simulink model "mchp_acim_dsPIC33A"  (R2025b)
settings: Solver=FixedStepDiscrete  StartTime=0.0  StopTime=25  FixedStep=Ts  RelTol=1e-3  EnableMultiTasking=on
values from neighbouring files (symbols this model uses):
  dataType = 'single'    [mchp_acim_foc_dsPIC33A_data.m]
  PWM_frequency = 20e3    (= 20000)    [mchp_acim_foc_dsPIC33A_data.m]
  PWM_frequency_mc = PWM_frequency    (= 20000)    [mchp_acim_foc_dsPIC33A_data.m]
  SpeedFilterCutoff = 40    [mchp_acim_foc_dsPIC33A_data.m]
  Ts = T_pwm    (= 5e-05)    [mchp_acim_foc_dsPIC33A_data.m]
  Ts_mc = T_pwm_mc    (= 5e-05)    [mchp_acim_foc_dsPIC33A_data.m]
  Ts_motor = T_pwm_mc    (= 5e-05)    [mchp_acim_foc_dsPIC33A_data.m]
  Ts_serialIn = 100e-3    (= 0.1)    [mchp_acim_foc_dsPIC33A_data.m]
undefined symbols (not defined in the file or in its folder): A0, A4, acim, ADC, appState, B0, C10, C11, C6, C7, C8, CS_param, D11, D12, DiscIntNeverNeededParam, estim_pll, estim_qei, inverter, Max, MaxPer, ms, NumBits1, NumBits2, P1, P17, P20, P39, P40, P41, P43, P44, P60, P61, PI_params_SI, Pin, PWM4_Trg1, Resol, s, target, us, VmaxPhase
libraries: simulink x47, MCHP_Blockset x24, mcbcontrolslib x5, mcbeeMathTransformLib x4, slpidlib x4, svdutilitieslib x1, autolibim x1, mcbplantlib x1
(part 4 of 6)

== system mchp_acim_dsPIC33A/MCHV-230VAC-1.5kW Development Board dsPIC33AK128MC106 MC DIM/ADC ==
  ADC HS 12b dsPICA : MCHP_Blockset/Analog IO/ADC HS 12b dsPICA  ADCREF=ADC 1 and ADC 2  ADC1_refChannel=0 (highest priority)  ADC2_refChannel=0 (highest priority)  ADC3_refChannel=Not used  ADC4_refChannel=Not used  ADC5_refChannel=Not used  CALRATE=once at startup  VREF_RNG=3.0V to 3.6V  BUFEN=off  info=0  SampleTime=1/Switching_Frequency  MCHP_PORT={ADC1_seq0.0}{ADC1A7}15:2:A7;{ADC2_seq0.0}{ADC2B7}15:2:B7;{ADC1_seq0.1}{ADC1B6}15:2:B6;{ADC1_seq0.0}{ADC1A7}15:2:A7;{ADC2_seq0.0}{ADC2B7}15:2:B7;{ADC1_seq0.1}{ADC1B6}15:2:B6;  MCHP_MASTERLINK=mchp_acim_dsPIC33A/MCHV-230VAC-1.5kW Development Board dsPIC33AK128MC106 MC DIM/Microchip Master  MCHP_CRC=33524962  ADC_Synchronisation=Triggered by custom source  ADC_Trig_TXT=PWM4_Trg1  ADC_TrigTimeStep=on  TrigSource_seq0_TXT=PWM4 adc trig 1  SampleTime_seq0_Tad_TXT="8.5 Tad  = 106ns  -  Rin < 11 kOhm"  ADC1_seq0_TXT=AD1 AN6 / A7 / Pin[2]  ADC1_seq0_align=Left aligned  ADC1_seq0_overSampling=x1 (12 bits)  ADC2_seq0_TXT=AD2 AN8 / B7 / Pin[30]  ADC2_seq0_align=Right aligned  ADC2_seq0_overSampling=x1 (12 bits)  ADC3_seq0_TXT="AD2 AN1 / B0 / Pin[20]  (L)"  ADC3_seq0_align=Right aligned  ADC3_seq0_overSampling=x1 (12 bits)  ADC4_seq0_TXT="AD2 AN1 / B0 / Pin[20]  (L)"  ADC4_seq0_align=Right aligned  ADC4_seq0_overSampling=x1 (12 bits)  ADC5_seq0_TXT="AD2 AN1 / B0 / Pin[20]  (L)"  ADC5_seq0_align=Right aligned  ADC5_seq0_overSampling=x1 (12 bits)  ADC1_seq0_1_TXT=AD1 AN8 / B6 / Pin[29]  ADC1_seq0_1_align=Left aligned  ADC1_seq0_1_overSampling=x1 (12 bits)  ADC2_seq0_1_TXT=Not Used  ADC2_seq0_1_align=Right aligned  ADC2_seq0_1_overSampling=x1 (12 bits)  ADC3_seq0_1_TXT=Not Used  ADC3_seq0_1_align=Right aligned  ADC3_seq0_1_overSampling=x1 (12 bits)  ADC4_seq0_1_TXT=Not Used  ADC4_seq0_1_align=Right aligned  ADC4_seq0_1_overSampling=x1 (12 bits)  ADC5_seq0_1_TXT=Not Used  ADC5_seq0_1_align=Right aligned  ADC5_seq0_1_overSampling=x1 (12 bits)  ADC1_seq0_2_TXT=Not Used  ADC1_seq0_2_align=Right aligned  ADC1_seq0_2_overSampling=x1 (12 bits)  ADC2_seq0_2_TXT=Not Used  ADC2_seq0_2_align=Right aligned  ADC2_seq0_2_overSampling=x1 (12 bits)  ADC3_seq0_2_TXT=Not Used  ADC3_seq0_2_align=Right aligned  ADC3_seq0_2_overSampling=x1 (12 bits)  ADC4_seq0_2_TXT=Not Used  ADC4_seq0_2_align=Right aligned  ADC4_seq0_2_overSampling=x1 (12 bits)  ADC5_seq0_2_TXT=Not Used  ADC5_seq0_2_align=Right aligned  ADC5_seq0_2_overSampling=x1 (12 bits)  ADC1_seq0_3_TXT=Not Used  ADC1_seq0_3_align=Right aligned  ADC1_seq0_3_overSampling=x1 (12 bits)  ADC2_seq0_3_TXT=Not Used  ADC2_seq0_3_align=Right aligned  ADC2_seq0_3_overSampling=x1 (12 bits)  ADC3_seq0_3_TXT=Not Used  ADC3_seq0_3_align=Right aligned  ADC3_seq0_3_overSampling=x1 (12 bits)  ADC4_seq0_3_TXT=Not Used  ADC4_seq0_3_align=Right aligned  ADC4_seq0_3_overSampling=x1 (12 bits)  ADC5_seq0_3_TXT=Not Used  ADC5_seq0_3_align=Right aligned  ADC5_seq0_3_overSampling=x1 (12 bits)  ADC1_seq0_4_TXT=Not Used  ADC1_seq0_4_align=Right aligned  ADC1_seq0_4_overSampling=x1 (12 bits)  ADC2_seq0_4_TXT=Not Used  ADC2_seq0_4_align=Right aligned  ADC2_seq0_4_overSampling=x1 (12 bits)  ADC3_seq0_4_TXT=Not Used  ADC3_seq0_4_align=Right aligned  ADC3_seq0_4_overSampling=x1 (12 bits)  ADC4_seq0_4_TXT=Not Used  ADC4_seq0_4_align=Right aligned  ADC4_seq0_4_overSampling=x1 (12 bits)  ADC5_seq0_4_TXT=Not Used  ADC5_seq0_4_align=Right aligned  ADC5_seq0_4_overSampling=x1 (12 bits)  ADC1_seq0_5_TXT=Not Used  ADC1_seq0_5_align=Right aligned  ADC1_seq0_5_overSampling=x1 (12 bits)  ADC2_seq0_5_TXT=Not Used  ADC2_seq0_5_align=Right aligned  ADC2_seq0_5_overSampling=x1 (12 bits)  ADC3_seq0_5_TXT=Not Used  ADC3_seq0_5_align=Right aligned  ADC3_seq0_5_overSampling=x1 (12 bits)  ADC4_seq0_5_TXT=Not Used  ADC4_seq0_5_align=Right aligned  ADC4_seq0_5_overSampling=x1 (12 bits)  ADC5_seq0_5_TXT=Not Used  ADC5_seq0_5_align=Right aligned  ADC5_seq0_5_overSampling=x1 (12 bits)  ADC_TRG2_ACCBRST_seq0=Burst - not interruptible  ADC1_NINSEL_seq0_TXT=Vss - single ended (unsigned)  ADC2_NINSEL_seq0_TXT=Vss - single ended (unsigned)  ADC3_NINSEL_seq0_TXT=Vss - single ended (unsigned)  ADC4_NINSEL_seq0_TXT=Vss - single ended (unsigned)  ADC5_NINSEL_seq0_TXT=Vss - single ended (unsigned)  TrigTimeStep_seq0=on  info_seq0=0  TrigSource_seq1_TXT=after previous sequence  SampleTime_seq1_Tad_TXT="4.5 Tad  = 56.2ns  -  Rin < 5.2 kOhm"  ADC1_seq1_TXT=Not Used  ADC1_seq1_align=Left aligned  ADC1_seq1_overSampling=x1 (12 bits)  ADC2_seq1_TXT=Not Used  ADC2_seq1_align=Right aligned  ADC2_seq1_overSampling=x1 (12 bits)  ADC3_seq1_TXT="AD2 AN1 / B0 / Pin[20]  (L)"  ADC3_seq1_align=Right aligned  ADC3_seq1_overSampling=x1 (12 bits)  ADC4_seq1_TXT="AD2 AN1 / B0 / Pin[20]  (L)"  ADC4_seq1_align=Right aligned  ADC4_seq1_overSampling=x1 (12 bits)  ADC5_seq1_TXT="AD2 AN1 / B0 / Pin[20]  (L)"  ADC5_seq1_align=Right aligned  ADC5_seq1_overSampling=x1 (12 bits)  ADC1_seq1_1_TXT=Not Used  ADC1_seq1_1_align=Right aligned  ADC1_seq1_1_overSampling=x1 (12 bits)  ADC2_seq1_1_TXT=Not Used  ADC2_seq1_1_align=Right aligned  ADC2_seq1_1_overSampling=x1 (12 bits)  ADC3_seq1_1_TXT=Not Used  ADC3_seq1_1_align=Right aligned  ADC3_seq1_1_overSampling=x1 (12 bits)  ADC4_seq1_1_TXT=Not Used  ADC4_seq1_1_align=Right aligned  ADC4_seq1_1_overSampling=x1 (12 bits)  ADC5_seq1_1_TXT=Not Used  ADC5_seq1_1_align=Right aligned  ADC5_seq1_1_overSampling=x1 (12 bits)  ADC1_seq1_2_TXT=Not Used  ADC1_seq1_2_align=Right aligned  ADC1_seq1_2_overSampling=x1 (12 bits)  ADC2_seq1_2_TXT=Not Used  ADC2_seq1_2_align=Right aligned  ADC2_seq1_2_overSampling=x1 (12 bits)  ADC3_seq1_2_TXT=Not Used  ADC3_seq1_2_align=Right aligned  ADC3_seq1_2_overSampling=x1 (12 bits)  ADC4_seq1_2_TXT=Not Used  ADC4_seq1_2_align=Right aligned  ADC4_seq1_2_overSampling=x1 (12 bits)  ADC5_seq1_2_TXT=Not Used  ADC5_seq1_2_align=Right aligned  ADC5_seq1_2_overSampling=x1 (12 bits)  ADC1_seq1_3_TXT=Not Used  ADC1_seq1_3_align=Right aligned  ADC1_seq1_3_overSampling=x1 (12 bits)  ADC2_seq1_3_TXT=Not Used  ADC2_seq1_3_align=Right aligned  ADC2_seq1_3_overSampling=x1 (12 bits)  ADC3_seq1_3_TXT=Not Used  ADC3_seq1_3_align=Right aligned  ADC3_seq1_3_overSampling=x1 (12 bits)  ADC4_seq1_3_TXT=Not Used  ADC4_seq1_3_align=Right aligned  ADC4_seq1_3_overSampling=x1 (12 bits)  ADC5_seq1_3_TXT=Not Used  ADC5_seq1_3_align=Right aligned  ADC5_seq1_3_overSampling=x1 (12 bits)  ADC1_seq1_4_TXT=Not Used  ADC1_seq1_4_align=Right aligned  ADC1_seq1_4_overSampling=x1 (12 bits)  ADC2_seq1_4_TXT=Not Used  ADC2_seq1_4_align=Right aligned  ADC2_seq1_4_overSampling=x1 (12 bits)  ADC3_seq1_4_TXT=Not Used  ADC3_seq1_4_align=Right aligned  ADC3_seq1_4_overSampling=x1 (12 bits)  ADC4_seq1_4_TXT=Not Used  ADC4_seq1_4_align=Right aligned  ADC4_seq1_4_overSampling=x1 (12 bits)  ADC5_seq1_4_TXT=Not Used  ADC5_seq1_4_align=Right aligned  ADC5_seq1_4_overSampling=x1 (12 bits)  ADC1_seq1_5_TXT=Not Used  ADC1_seq1_5_align=Right aligned  ADC1_seq1_5_overSampling=x1 (12 bits)  ADC2_seq1_5_TXT=Not Used  ADC2_seq1_5_align=Right aligned  ADC2_seq1_5_overSampling=x1 (12 bits)  ADC3_seq1_5_TXT=Not Used  ADC3_seq1_5_align=Right aligned  ADC3_seq1_5_overSampling=x1 (12 bits)  ADC4_seq1_5_TXT=Not Used  ADC4_seq1_5_align=Right aligned  ADC4_seq1_5_overSampling=x1 (12 bits)  ADC5_seq1_5_TXT=Not Used  ADC5_seq1_5_align=Right aligned  ADC5_seq1_5_overSampling=x1 (12 bits)  ADC_TRG2_ACCBRST_seq1=Burst - not interruptible  ADC1_NINSEL_seq1_TXT=Vss - single ended (unsigned)  ADC2_NINSEL_seq1_TXT=Vss - single ended (unsigned)  ADC3_NINSEL_seq1_TXT=Vss - single ended (unsigned)  ADC4_NINSEL_seq1_TXT=Vss - single ended (unsigned)  ADC5_NINSEL_seq1_TXT=Vss - single ended (unsigned)  TrigTimeStep_seq1=on  info_seq1=0  TrigSource_seq2_TXT=after previous sequence  SampleTime_seq2_Tad_TXT="4.5 Tad  = 56.2ns  -  Rin < 5.2 kOhm"  ADC1_seq2_TXT=Not Used  ADC1_seq2_align=Left aligned  ADC1_seq2_overSampling=x1 (12 bits)  ADC2_seq2_TXT=Not Used  ADC2_seq2_align=Right aligned  ADC2_seq2_overSampling=x1 (12 bits)  ADC3_seq2_TXT="AD2 AN1 / B0 / Pin[20]  (L)"  ADC3_seq2_align=Right aligned  ADC3_seq2_overSampling=x1 (12 bits)  ADC4_seq2_TXT="AD2 AN1 / B0 / Pin[20]  (L)"  ADC4_seq2_align=Right aligned  ADC4_seq2_overSampling=x1 (12 bits)  ADC5_seq2_TXT="AD2 AN1 / B0 / Pin[20]  (L)"  ADC5_seq2_align=Right aligned  ADC5_seq2_overSampling=x1 (12 bits)  ADC1_seq2_1_TXT=Not Used  ADC1_seq2_1_align=Right aligned  ADC1_seq2_1_overSampling=x1 (12 bits)  ADC2_seq2_1_TXT=Not Used  ADC2_seq2_1_align=Right aligned  ADC2_seq2_1_overSampling=x1 (12 bits)  ADC3_seq2_1_TXT=Not Used  ADC3_seq2_1_align=Right aligned  ADC3_seq2_1_overSampling=x1 (12 bits)  ADC4_seq2_1_TXT=Not Used  ADC4_seq2_1_align=Right aligned  ADC4_seq2_1_overSampling=x1 (12 bits)  ADC5_seq2_1_TXT=Not Used  ADC5_seq2_1_align=Right aligned  ADC5_seq2_1_overSampling=x1 (12 bits)  ADC1_seq2_2_TXT=Not Used  ADC1_seq2_2_align=Right aligned  ADC1_seq2_2_overSampling=x1 (12 bits)  ADC2_seq2_2_TXT=Not Used  ADC2_seq2_2_align=Right aligned  ADC2_seq2_2_overSampling=x1 (12 bits)  ADC3_seq2_2_TXT=Not Used  ADC3_seq2_2_align=Right aligned  ADC3_seq2_2_overSampling=x1 (12 bits)  ADC4_seq2_2_TXT=Not Used  ADC4_seq2_2_align=Right aligned  ADC4_seq2_2_overSampling=x1 (12 bits)  ADC5_seq2_2_TXT=Not Used  ADC5_seq2_2_align=Right aligned  ADC5_seq2_2_overSampling=x1 (12 bits)  ADC1_seq2_3_TXT=Not Used  ADC1_seq2_3_align=Right aligned  ADC1_seq2_3_overSampling=x1 (12 bits)  ADC2_seq2_3_TXT=Not Used  ADC2_seq2_3_align=Right aligned  ADC2_seq2_3_overSampling=x1 (12 bits)  ADC3_seq2_3_TXT=Not Used  ADC3_seq2_3_align=Right aligned  ADC3_seq2_3_overSampling=x1 (12 bits)  ADC4_seq2_3_TXT=Not Used  ADC4_seq2_3_align=Right aligned  ADC4_seq2_3_overSampling=x1 (12 bits)  ADC5_seq2_3_TXT=Not Used  ADC5_seq2_3_align=Right aligned  ADC5_seq2_3_overSampling=x1 (12 bits)  ADC1_seq2_4_TXT=Not Used  ADC1_seq2_4_align=Right aligned  ADC1_seq2_4_overSampling=x1 (12 bits)  ADC2_seq2_4_TXT=Not Used  ADC2_seq2_4_align=Right aligned  ADC2_seq2_4_overSampling=x1 (12 bits)  ADC3_seq2_4_TXT=Not Used  ADC3_seq2_4_align=Right aligned  ADC3_seq2_4_overSampling=x1 (12 bits)  ADC4_seq2_4_TXT=Not Used  ADC4_seq2_4_align=Right aligned  ADC4_seq2_4_overSampling=x1 (12 bits)  ADC5_seq2_4_TXT=Not Used  ADC5_seq2_4_align=Right aligned  ADC5_seq2_4_overSampling=x1 (12 bits)  ADC1_seq2_5_TXT=Not Used  ADC1_seq2_5_align=Right aligned  ADC1_seq2_5_overSampling=x1 (12 bits)  ADC2_seq2_5_TXT=Not Used  ADC2_seq2_5_align=Right aligned  ADC2_seq2_5_overSampling=x1 (12 bits)  ADC3_seq2_5_TXT=Not Used  ADC3_seq2_5_align=Right aligned  ADC3_seq2_5_overSampling=x1 (12 bits)  ADC4_seq2_5_TXT=Not Used  ADC4_seq2_5_align=Right aligned  ADC4_seq2_5_overSampling=x1 (12 bits)  ADC5_seq2_5_TXT=Not Used  ADC5_seq2_5_align=Right aligned  ADC5_seq2_5_overSampling=x1 (12 bits)  ADC_TRG2_ACCBRST_seq2=Burst - not interruptible  ADC1_NINSEL_seq2_TXT=Vss - single ended (unsigned)  ADC2_NINSEL_seq2_TXT=Vss - single ended (unsigned)  ADC3_NINSEL_seq2_TXT=Vss - single ended (unsigned)  ADC4_NINSEL_seq2_TXT=Vss - single ended (unsigned)  ADC5_NINSEL_seq2_TXT=Vss - single ended (unsigned)  TrigTimeStep_seq2=on  info_seq2=0  TrigSource_seq3_TXT=after previous sequence  SampleTime_seq3_Tad_TXT="4.5 Tad  = 56.2ns  -  Rin < 5.2 kOhm"  ADC1_seq3_TXT=Not Used  ADC1_seq3_align=Left aligned  ADC1_seq3_overSampling=x1 (12 bits)  ADC2_seq3_TXT=Not Used  ADC2_seq3_align=Right aligned  ADC2_seq3_overSampling=x1 (12 bits)  ADC3_seq3_TXT="AD2 AN1 / B0 / Pin[20]  (L)"  ADC3_seq3_align=Right aligned  ADC3_seq3_overSampling=x1 (12 bits)  ADC4_seq3_TXT="AD2 AN1 / B0 / Pin[20]  (L)"  ADC4_seq3_align=Right aligned  ADC4_seq3_overSampling=x1 (12 bits)  ADC5_seq3_TXT="AD2 AN1 / B0 / Pin[20]  (L)"  ADC5_seq3_align=Right aligned  ADC5_seq3_overSampling=x1 (12 bits)  ADC1_seq3_1_TXT=Not Used  ADC1_seq3_1_align=Right aligned  ADC1_seq3_1_overSampling=x1 (12 bits)  ADC2_seq3_1_TXT=Not Used  ADC2_seq3_1_align=Right aligned  ADC2_seq3_1_overSampling=x1 (12 bits)  ADC3_seq3_1_TXT=Not Used  ADC3_seq3_1_align=Right aligned  ADC3_seq3_1_overSampling=x1 (12 bits)  ADC4_seq3_1_TXT=Not Used  ADC4_seq3_1_align=Right aligned  ADC4_seq3_1_overSampling=x1 (12 bits)  ADC5_seq3_1_TXT=Not Used  ADC5_seq3_1_align=Right aligned  ADC5_seq3_1_overSampling=x1 (12 bits)  ADC1_seq3_2_TXT=Not Used  ADC1_seq3_2_align=Right aligned  ADC1_seq3_2_overSampling=x1 (12 bits)  ADC2_seq3_2_TXT=Not Used  ADC2_seq3_2_align=Right aligned  ADC2_seq3_2_overSampling=x1 (12 bits)  ADC3_seq3_2_TXT=Not Used  ADC3_seq3_2_align=Right aligned  ADC3_seq3_2_overSampling=x1 (12 bits)  ADC4_seq3_2_TXT=Not Used  ADC4_seq3_2_align=Right aligned  ADC4_seq3_2_overSampling=x1 (12 bits)  ADC5_seq3_2_TXT=Not Used  ADC5_seq3_2_align=Right aligned  ADC5_seq3_2_overSampling=x1 (12 bits)  ADC1_seq3_3_TXT=Not Used  ADC1_seq3_3_align=Right aligned  ADC1_seq3_3_overSampling=x1 (12 bits)  ADC2_seq3_3_TXT=Not Used  ADC2_seq3_3_align=Right aligned  ADC2_seq3_3_overSampling=x1 (12 bits)  ADC3_seq3_3_TXT=Not Used  ADC3_seq3_3_align=Right aligned  ADC3_seq3_3_overSampling=x1 (12 bits)  ADC4_seq3_3_TXT=Not Used  ADC4_seq3_3_align=Right aligned  ADC4_seq3_3_overSampling=x1 (12 bits)  ADC5_seq3_3_TXT=Not Used  ADC5_seq3_3_align=Right aligned  ADC5_seq3_3_overSampling=x1 (12 bits)  ADC1_seq3_4_TXT=Not Used  ADC1_seq3_4_align=Right aligned  ADC1_seq3_4_overSampling=x1 (12 bits)  ADC2_seq3_4_TXT=Not Used  ADC2_seq3_4_align=Right aligned  ADC2_seq3_4_overSampling=x1 (12 bits)  ADC3_seq3_4_TXT=Not Used  ADC3_seq3_4_align=Right aligned  ADC3_seq3_4_overSampling=x1 (12 bits)  ADC4_seq3_4_TXT=Not Used  ADC4_seq3_4_align=Right aligned  ADC4_seq3_4_overSampling=x1 (12 bits)  ADC5_seq3_4_TXT=Not Used  ADC5_seq3_4_align=Right aligned  ADC5_seq3_4_overSampling=x1 (12 bits)  ADC1_seq3_5_TXT=Not Used  ADC1_seq3_5_align=Right aligned  ADC1_seq3_5_overSampling=x1 (12 bits)  ADC2_seq3_5_TXT=Not Used  ADC2_seq3_5_align=Right aligned  ADC2_seq3_5_overSampling=x1 (12 bits)  ADC3_seq3_5_TXT=Not Used  ADC3_seq3_5_align=Right aligned  ADC3_seq3_5_overSampling=x1 (12 bits)  ADC4_seq3_5_TXT=Not Used  ADC4_seq3_5_align=Right aligned  ADC4_seq3_5_overSampling=x1 (12 bits)  ADC5_seq3_5_TXT=Not Used  ADC5_seq3_5_align=Right aligned  ADC5_seq3_5_overSampling=x1 (12 bits)  ADC_TRG2_ACCBRST_seq3=Burst - not interruptible  ADC1_NINSEL_seq3_TXT=Vss - single ended (unsigned)  ADC2_NINSEL_seq3_TXT=Vss - single ended (unsigned)  ADC3_NINSEL_seq3_TXT=Vss - single ended (unsigned)  ADC4_NINSEL_seq3_TXT=Vss - single ended (unsigned)  ADC5_NINSEL_seq3_TXT=Vss - single ended (unsigned)  TrigTimeStep_seq3=on  info_seq3=0  TrigSource_seq4_TXT=after previous sequence  SampleTime_seq4_Tad_TXT="4.5 Tad  = 56.2ns  -  Rin < 5.2 kOhm"  ADC1_seq4_TXT=Not Used  ADC1_seq4_align=Left aligned  ADC1_seq4_overSampling=x1 (12 bits)  ADC2_seq4_TXT=Not Used  ADC2_seq4_align=Right aligned  ADC2_seq4_overSampling=x1 (12 bits)  ADC3_seq4_TXT="AD2 AN1 / B0 / Pin[20]  (L)"  ADC3_seq4_align=Right aligned  ADC3_seq4_overSampling=x1 (12 bits)  ADC4_seq4_TXT="AD2 AN1 / B0 / Pin[20]  (L)"  ADC4_seq4_align=Right aligned  ADC4_seq4_overSampling=x1 (12 bits)  ADC5_seq4_TXT="AD2 AN1 / B0 / Pin[20]  (L)"  ADC5_seq4_align=Right aligned  ADC5_seq4_overSampling=x1 (12 bits)  ADC1_seq4_1_TXT=Not Used  ADC1_seq4_1_align=Right aligned  ADC1_seq4_1_overSampling=x1 (12 bits)  ADC2_seq4_1_TXT=Not Used  ADC2_seq4_1_align=Right aligned  ADC2_seq4_1_overSampling=x1 (12 bits)  ADC3_seq4_1_TXT=Not Used  ADC3_seq4_1_align=Right aligned  ADC3_seq4_1_overSampling=x1 (12 bits)  ADC4_seq4_1_TXT=Not Used  ADC4_seq4_1_align=Right aligned  ADC4_seq4_1_overSampling=x1 (12 bits)  ADC5_seq4_1_TXT=Not Used  ADC5_seq4_1_align=Right aligned  ADC5_seq4_1_overSampling=x1 (12 bits)  ADC1_seq4_2_TXT=Not Used  ADC1_seq4_2_align=Right aligned  ADC1_seq4_2_overSampling=x1 (12 bits)  ADC2_seq4_2_TXT=Not Used  ADC2_seq4_2_align=Right aligned  ADC2_seq4_2_overSampling=x1 (12 bits)  ADC3_seq4_2_TXT=Not Used  ADC3_seq4_2_align=Right aligned  ADC3_seq4_2_overSampling=x1 (12 bits)  ADC4_seq4_2_TXT=Not Used  ADC4_seq4_2_align=Right aligned  ADC4_seq4_2_overSampling=x1 (12 bits)  ADC5_seq4_2_TXT=Not Used  ADC5_seq4_2_align=Right aligned  ADC5_seq4_2_overSampling=x1 (12 bits)  ADC1_seq4_3_TXT=Not Used  ADC1_seq4_3_align=Right aligned  ADC1_seq4_3_overSampling=x1 (12 bits)  ADC2_seq4_3_TXT=Not Used  ADC2_seq4_3_align=Right aligned  ADC2_seq4_3_overSampling=x1 (12 bits)  ADC3_seq4_3_TXT=Not Used  ADC3_seq4_3_align=Right aligned  ADC3_seq4_3_overSampling=x1 (12 bits)  ADC4_seq4_3_TXT=Not Used  ADC4_seq4_3_align=Right aligned  ADC4_seq4_3_overSampling=x1 (12 bits)  ADC5_seq4_3_TXT=Not Used  ADC5_seq4_3_align=Right aligned  ADC5_seq4_3_overSampling=x1 (12 bits)  ADC1_seq4_4_TXT=Not Used  ADC1_seq4_4_align=Right aligned  ADC1_seq4_4_overSampling=x1 (12 bits)  ADC2_seq4_4_TXT=Not Used  ADC2_seq4_4_align=Right aligned  ADC2_seq4_4_overSampling=x1 (12 bits)  ADC3_seq4_4_TXT=Not Used  ADC3_seq4_4_align=Right aligned  ADC3_seq4_4_overSampling=x1 (12 bits)  ADC4_seq4_4_TXT=Not Used  ADC4_seq4_4_align=Right aligned  ADC4_seq4_4_overSampling=x1 (12 bits)  ADC5_seq4_4_TXT=Not Used  ADC5_seq4_4_align=Right aligned  ADC5_seq4_4_overSampling=x1 (12 bits)  ADC1_seq4_5_TXT=Not Used  ADC1_seq4_5_align=Right aligned  ADC1_seq4_5_overSampling=x1 (12 bits)  ADC2_seq4_5_TXT=Not Used  ADC2_seq4_5_align=Right aligned  ADC2_seq4_5_overSampling=x1 (12 bits)  ADC3_seq4_5_TXT=Not Used  ADC3_seq4_5_align=Right aligned  ADC3_seq4_5_overSampling=x1 (12 bits)  ADC4_seq4_5_TXT=Not Used  ADC4_seq4_5_align=Right aligned  ADC4_seq4_5_overSampling=x1 (12 bits)  ADC5_seq4_5_TXT=Not Used  ADC5_seq4_5_align=Right aligned  ADC5_seq4_5_overSampling=x1 (12 bits)  ADC_TRG2_ACCBRST_seq4=Burst - not interruptible  ADC1_NINSEL_seq4_TXT=Vss - single ended (unsigned)  ADC2_NINSEL_seq4_TXT=Vss - single ended (unsigned)  ADC3_NINSEL_seq4_TXT=Vss - single ended (unsigned)  ADC4_NINSEL_seq4_TXT=Vss - single ended (unsigned)  ADC5_NINSEL_seq4_TXT=Vss - single ended (unsigned)  TrigTimeStep_seq4=on  info_seq4=0  TrigSource_seq5_TXT=after previous sequence  SampleTime_seq5_Tad_TXT="4.5 Tad  = 56.2ns  -  Rin < 5.2 kOhm"  ADC1_seq5_TXT=Not Used  ADC1_seq5_align=Left aligned  ADC1_seq5_overSampling=x1 (12 bits)  ADC2_seq5_TXT=Not Used  ADC2_seq5_align=Right aligned  ADC2_seq5_overSampling=x1 (12 bits)  ADC3_seq5_TXT="AD2 AN1 / B0 / Pin[20]  (L)"  ADC3_seq5_align=Right aligned  ADC3_seq5_overSampling=x1 (12 bits)  ADC4_seq5_TXT="AD2 AN1 / B0 / Pin[20]  (L)"  ADC4_seq5_align=Right aligned  ADC4_seq5_overSampling=x1 (12 bits)  ADC5_seq5_TXT="AD2 AN1 / B0 / Pin[20]  (L)"  ADC5_seq5_align=Right aligned  ADC5_seq5_overSampling=x1 (12 bits)  ADC1_seq5_1_TXT=Not Used  ADC1_seq5_1_align=Right aligned  ADC1_seq5_1_overSampling=x1 (12 bits)  ADC2_seq5_1_TXT=Not Used  ADC2_seq5_1_align=Right aligned  ADC2_seq5_1_overSampling=x1 (12 bits)  ADC3_seq5_1_TXT=Not Used  ADC3_seq5_1_align=Right aligned  ADC3_seq5_1_overSampling=x1 (12 bits)  ADC4_seq5_1_TXT=Not Used  ADC4_seq5_1_align=Right aligned  ADC4_seq5_1_overSampling=x1 (12 bits)  ADC5_seq5_1_TXT=Not Used  ADC5_seq5_1_align=Right aligned  ADC5_seq5_1_overSampling=x1 (12 bits)  ADC1_seq5_2_TXT=Not Used  ADC1_seq5_2_align=Right aligned  ADC1_seq5_2_overSampling=x1 (12 bits)  ADC2_seq5_2_TXT=Not Used  ADC2_seq5_2_align=Right aligned  ADC2_seq5_2_overSampling=x1 (12 bits)  ADC3_seq5_2_TXT=Not Used  ADC3_seq5_2_align=Right aligned  ADC3_seq5_2_overSampling=x1 (12 bits)  ADC4_seq5_2_TXT=Not Used  ADC4_seq5_2_align=Right aligned  ADC4_seq5_2_overSampling=x1 (12 bits)  ADC5_seq5_2_TXT=Not Used  ADC5_seq5_2_align=Right aligned  ADC5_seq5_2_overSampling=x1 (12 bits)  ADC1_seq5_3_TXT=Not Used  ADC1_seq5_3_align=Right aligned  ADC1_seq5_3_overSampling=x1 (12 bits)  ADC2_seq5_3_TXT=Not Used  ADC2_seq5_3_align=Right aligned  ADC2_seq5_3_overSampling=x1 (12 bits)  ADC3_seq5_3_TXT=Not Used  ADC3_seq5_3_align=Right aligned  ADC3_seq5_3_overSampling=x1 (12 bits)  ADC4_seq5_3_TXT=Not Used  ADC4_seq5_3_align=Right aligned  ADC4_seq5_3_overSampling=x1 (12 bits)  ADC5_seq5_3_TXT=Not Used  ADC5_seq5_3_align=Right aligned  ADC5_seq5_3_overSampling=x1 (12 bits)  ADC1_seq5_4_TXT=Not Used  ADC1_seq5_4_align=Right aligned  ADC1_seq5_4_overSampling=x1 (12 bits)  ADC2_seq5_4_TXT=Not Used  ADC2_seq5_4_align=Right aligned  ADC2_seq5_4_overSampling=x1 (12 bits)  ADC3_seq5_4_TXT=Not Used  ADC3_seq5_4_align=Right aligned  ADC3_seq5_4_overSampling=x1 (12 bits)  ADC4_seq5_4_TXT=Not Used  ADC4_seq5_4_align=Right aligned  ADC4_seq5_4_overSampling=x1 (12 bits)  ADC5_seq5_4_TXT=Not Used  ADC5_seq5_4_align=Right aligned  ADC5_seq5_4_overSampling=x1 (12 bits)  ADC1_seq5_5_TXT=Not Used  ADC1_seq5_5_align=Right aligned  ADC1_seq5_5_overSampling=x1 (12 bits)  ADC2_seq5_5_TXT=Not Used  ADC2_seq5_5_align=Right aligned  ADC2_seq5_5_overSampling=x1 (12 bits)  ADC3_seq5_5_TXT=Not Used  ADC3_seq5_5_align=Right aligned  ADC3_seq5_5_overSampling=x1 (12 bits)  ADC4_seq5_5_TXT=Not Used  ADC4_seq5_5_align=Right aligned  ADC4_seq5_5_overSampling=x1 (12 bits)  ADC5_seq5_5_TXT=Not Used  ADC5_seq5_5_align=Right aligned  ADC5_seq5_5_overSampling=x1 (12 bits)  ADC_TRG2_ACCBRST_seq5=Burst - not interruptible  ADC1_NINSEL_seq5_TXT=Vss - single ended (unsigned)  ADC2_NINSEL_seq5_TXT=Vss - single ended (unsigned)  ADC3_NINSEL_seq5_TXT=Vss - single ended (unsigned)  ADC4_NINSEL_seq5_TXT=Vss - single ended (unsigned)  ADC5_NINSEL_seq5_TXT=Vss - single ended (unsigned)  TrigTimeStep_seq5=on  info_seq5=0
      settings: SourceProductName=MPLAB Device Blocks for Simulink
  ADC HS 12b dsPICA1 : MCHP_Blockset/Analog IO/ADC HS 12b dsPICA  ADCREF=ADC 1 and ADC 2  ADC1_refChannel=5  ADC2_refChannel=5  ADC3_refChannel=Not used  ADC4_refChannel=Not used  ADC5_refChannel=Not used  CALRATE=once at startup  VREF_RNG=3.0V to 3.6V  BUFEN=off  info=0  SampleTime=1/Switching_Frequency_MC  MCHP_PORT={ADC1_seq0.0}{ADC1A2}15:2:A2;{ADC2_seq0.0}{ADC2B0}15:2:B0;{ADC1_seq0.1}{ADC1A11}15:2:A11;{ADC1_seq0.2}{ADC1A5}15:2:A5;{ADC2_seq0.2}{ADC2A8}15:2:A8;{ADC1_seq0.0}{ADC1A2}15:2:A2;{ADC2_seq0.0}{ADC2B0}15:2:B0;{ADC1_seq0.1}{ADC1A11}15:2:A11;{ADC1_seq0.2}{ADC1A5}15:2:A5;{ADC2_seq0.2}{ADC2A8}15:2:A8;  MCHP_MASTERLINK=mchp_acim_dsPIC33A/MCHV-230VAC-1.5kW Development Board dsPIC33AK128MC106 MC DIM/Microchip Master  MCHP_CRC=33977867  ADC_Synchronisation=off  ADC_Trig_TXT=off  ADC_TrigTimeStep=off  TrigSource_seq0_TXT=PWM1 adc trig 1  SampleTime_seq0_Tad_TXT="4.5 Tad  = 56.2ns  -  Rin < 5.2 kOhm"  ADC1_seq0_TXT=AD1 AN0 / A2 / Pin[12]  ADC1_seq0_align=Left aligned  ADC1_seq0_overSampling=x1 (12 bits)  ADC2_seq0_TXT=AD2 AN1 / B0 / Pin[20]  ADC2_seq0_align=Left aligned  ADC2_seq0_overSampling=x1 (12 bits)  ADC3_seq0_TXT="AD2 AN1 / B0 / Pin[20]  (L)"  ADC3_seq0_align=Right aligned  ADC3_seq0_overSampling=x1 (12 bits)  ADC4_seq0_TXT="AD2 AN1 / B0 / Pin[20]  (L)"  ADC4_seq0_align=Right aligned  ADC4_seq0_overSampling=x1 (12 bits)  ADC5_seq0_TXT="AD2 AN1 / B0 / Pin[20]  (L)"  ADC5_seq0_align=Right aligned  ADC5_seq0_overSampling=x1 (12 bits)  ADC1_seq0_1_TXT=AD1 AN10 / A11 / Pin[6]  ADC1_seq0_1_align=Left aligned  ADC1_seq0_1_overSampling=x1 (12 bits)  ADC2_seq0_1_TXT=Not Used  ADC2_seq0_1_align=Left aligned  ADC2_seq0_1_overSampling=x1 (12 bits)  ADC3_seq0_1_TXT=Not Used  ADC3_seq0_1_align=Right aligned  ADC3_seq0_1_overSampling=x1 (12 bits)  ADC4_seq0_1_TXT=Not Used  ADC4_seq0_1_align=Right aligned  ADC4_seq0_1_overSampling=x1 (12 bits)  ADC5_seq0_1_TXT=Not Used  ADC5_seq0_1_align=Right aligned  ADC5_seq0_1_overSampling=x1 (12 bits)  ADC1_seq0_2_TXT=AD1 AN3 / A5 / Pin[15]  ADC1_seq0_2_align=Right aligned  ADC1_seq0_2_overSampling=x1 (12 bits)  ADC2_seq0_2_TXT=AD2 AN9 / A8 / Pin[7]  ADC2_seq0_2_align=Right aligned  ADC2_seq0_2_overSampling=x1 (12 bits)  ADC3_seq0_2_TXT=Not Used  ADC3_seq0_2_align=Right aligned  ADC3_seq0_2_overSampling=x1 (12 bits)  ADC4_seq0_2_TXT=Not Used  ADC4_seq0_2_align=Right aligned  ADC4_seq0_2_overSampling=x1 (12 bits)  ADC5_seq0_2_TXT=Not Used  ADC5_seq0_2_align=Right aligned  ADC5_seq0_2_overSampling=x1 (12 bits)  ADC1_seq0_3_TXT=Not Used  ADC1_seq0_3_align=Right aligned  ADC1_seq0_3_overSampling=x1 (12 bits)  ADC2_seq0_3_TXT=Not Used  ADC2_seq0_3_align=Right aligned  ADC2_seq0_3_overSampling=x1 (12 bits)  ADC3_seq0_3_TXT=Not Used  ADC3_seq0_3_align=Right aligned  ADC3_seq0_3_overSampling=x1 (12 bits)  ADC4_seq0_3_TXT=Not Used  ADC4_seq0_3_align=Right aligned  ADC4_seq0_3_overSampling=x1 (12 bits)  ADC5_seq0_3_TXT=Not Used  ADC5_seq0_3_align=Right aligned  ADC5_seq0_3_overSampling=x1 (12 bits)  ADC1_seq0_4_TXT=Not Used  ADC1_seq0_4_align=Right aligned  ADC1_seq0_4_overSampling=x1 (12 bits)  ADC2_seq0_4_TXT=Not Used  ADC2_seq0_4_align=Right aligned  ADC2_seq0_4_overSampling=x1 (12 bits)  ADC3_seq0_4_TXT=Not Used  ADC3_seq0_4_align=Right aligned  ADC3_seq0_4_overSampling=x1 (12 bits)  ADC4_seq0_4_TXT=Not Used  ADC4_seq0_4_align=Right aligned  ADC4_seq0_4_overSampling=x1 (12 bits)  ADC5_seq0_4_TXT=Not Used  ADC5_seq0_4_align=Right aligned  ADC5_seq0_4_overSampling=x1 (12 bits)  ADC1_seq0_5_TXT=Not Used  ADC1_seq0_5_align=Right aligned  ADC1_seq0_5_overSampling=x1 (12 bits)  ADC2_seq0_5_TXT=Not Used  ADC2_seq0_5_align=Right aligned  ADC2_seq0_5_overSampling=x1 (12 bits)  ADC3_seq0_5_TXT=Not Used  ADC3_seq0_5_align=Right aligned  ADC3_seq0_5_overSampling=x1 (12 bits)  ADC4_seq0_5_TXT=Not Used  ADC4_seq0_5_align=Right aligned  ADC4_seq0_5_overSampling=x1 (12 bits)  ADC5_seq0_5_TXT=Not Used  ADC5_seq0_5_align=Right aligned  ADC5_seq0_5_overSampling=x1 (12 bits)  ADC_TRG2_ACCBRST_seq0=Burst - not interruptible  ADC1_NINSEL_seq0_TXT=Vss - single ended (unsigned)  ADC2_NINSEL_seq0_TXT=Vss - single ended (unsigned)  ADC3_NINSEL_seq0_TXT=Vss - single ended (unsigned)  ADC4_NINSEL_seq0_TXT=Vss - single ended (unsigned)  ADC5_NINSEL_seq0_TXT=Vss - single ended (unsigned)  TrigTimeStep_seq0=off  info_seq0=0  TrigSource_seq1_TXT=after previous sequence  SampleTime_seq1_Tad_TXT="0.5 Tad  = 6.25ns  -  Rin < 0 kOhm"  ADC1_seq1_TXT=Not Used  ADC1_seq1_align=Right aligned  ADC1_seq1_overSampling=x1 (12 bits)  ADC2_seq1_TXT=Not Used  ADC2_seq1_align=Right aligned  ADC2_seq1_overSampling=x1 (12 bits)  ADC3_seq1_TXT=Not Used  ADC3_seq1_align=Right aligned  ADC3_seq1_overSampling=x1 (12 bits)  ADC4_seq1_TXT=Not Used  ADC4_seq1_align=Right aligned  ADC4_seq1_overSampling=x1 (12 bits)  ADC5_seq1_TXT=Not Used  ADC5_seq1_align=Right aligned  ADC5_seq1_overSampling=x1 (12 bits)  ADC1_seq1_1_TXT=Not Used  ADC1_seq1_1_align=Right aligned  ADC1_seq1_1_overSampling=x1 (12 bits)  ADC2_seq1_1_TXT=Not Used  ADC2_seq1_1_align=Right aligned  ADC2_seq1_1_overSampling=x1 (12 bits)  ADC3_seq1_1_TXT=Not Used  ADC3_seq1_1_align=Right aligned  ADC3_seq1_1_overSampling=x1 (12 bits)  ADC4_seq1_1_TXT=Not Used  ADC4_seq1_1_align=Right aligned  ADC4_seq1_1_overSampling=x1 (12 bits)  ADC5_seq1_1_TXT=Not Used  ADC5_seq1_1_align=Right aligned  ADC5_seq1_1_overSampling=x1 (12 bits)  ADC1_seq1_2_TXT=Not Used  ADC1_seq1_2_align=Right aligned  ADC1_seq1_2_overSampling=x1 (12 bits)  ADC2_seq1_2_TXT=Not Used  ADC2_seq1_2_align=Right aligned  ADC2_seq1_2_overSampling=x1 (12 bits)  ADC3_seq1_2_TXT=Not Used  ADC3_seq1_2_align=Right aligned  ADC3_seq1_2_overSampling=x1 (12 bits)  ADC4_seq1_2_TXT=Not Used  ADC4_seq1_2_align=Right aligned  ADC4_seq1_2_overSampling=x1 (12 bits)  ADC5_seq1_2_TXT=Not Used  ADC5_seq1_2_align=Right aligned  ADC5_seq1_2_overSampling=x1 (12 bits)  ADC1_seq1_3_TXT=Not Used  ADC1_seq1_3_align=Right aligned  ADC1_seq1_3_overSampling=x1 (12 bits)  ADC2_seq1_3_TXT=Not Used  ADC2_seq1_3_align=Right aligned  ADC2_seq1_3_overSampling=x1 (12 bits)  ADC3_seq1_3_TXT=Not Used  ADC3_seq1_3_align=Right aligned  ADC3_seq1_3_overSampling=x1 (12 bits)  ADC4_seq1_3_TXT=Not Used  ADC4_seq1_3_align=Right aligned  ADC4_seq1_3_overSampling=x1 (12 bits)  ADC5_seq1_3_TXT=Not Used  ADC5_seq1_3_align=Right aligned  ADC5_seq1_3_overSampling=x1 (12 bits)  ADC1_seq1_4_TXT=Not Used  ADC1_seq1_4_align=Right aligned  ADC1_seq1_4_overSampling=x1 (12 bits)  ADC2_seq1_4_TXT=Not Used  ADC2_seq1_4_align=Right aligned  ADC2_seq1_4_overSampling=x1 (12 bits)  ADC3_seq1_4_TXT=Not Used  ADC3_seq1_4_align=Right aligned  ADC3_seq1_4_overSampling=x1 (12 bits)  ADC4_seq1_4_TXT=Not Used  ADC4_seq1_4_align=Right aligned  ADC4_seq1_4_overSampling=x1 (12 bits)  ADC5_seq1_4_TXT=Not Used  ADC5_seq1_4_align=Right aligned  ADC5_seq1_4_overSampling=x1 (12 bits)  ADC1_seq1_5_TXT=Not Used  ADC1_seq1_5_align=Right aligned  ADC1_seq1_5_overSampling=x1 (12 bits)  ADC2_seq1_5_TXT=Not Used  ADC2_seq1_5_align=Right aligned  ADC2_seq1_5_overSampling=x1 (12 bits)  ADC3_seq1_5_TXT=Not Used  ADC3_seq1_5_align=Right aligned  ADC3_seq1_5_overSampling=x1 (12 bits)  ADC4_seq1_5_TXT=Not Used  ADC4_seq1_5_align=Right aligned  ADC4_seq1_5_overSampling=x1 (12 bits)  ADC5_seq1_5_TXT=Not Used  ADC5_seq1_5_align=Right aligned  ADC5_seq1_5_overSampling=x1 (12 bits)  ADC_TRG2_ACCBRST_seq1=Burst - not interruptible  ADC1_NINSEL_seq1_TXT=Vss - single ended (unsigned)  ADC2_NINSEL_seq1_TXT=Vss - single ended (unsigned)  ADC3_NINSEL_seq1_TXT=Vss - single ended (unsigned)  ADC4_NINSEL_seq1_TXT=Vss - single ended (unsigned)  ADC5_NINSEL_seq1_TXT=Vss - single ended (unsigned)  TrigTimeStep_seq1=off  info_seq1=0  TrigSource_seq2_TXT=after previous sequence  SampleTime_seq2_Tad_TXT="0.5 Tad  = 6.25ns  -  Rin < 0 kOhm"  ADC1_seq2_TXT=Not Used  ADC1_seq2_align=Right aligned  ADC1_seq2_overSampling=x1 (12 bits)  ADC2_seq2_TXT=Not Used  ADC2_seq2_align=Right aligned  ADC2_seq2_overSampling=x1 (12 bits)  ADC3_seq2_TXT=Not Used  ADC3_seq2_align=Right aligned  ADC3_seq2_overSampling=x1 (12 bits)  ADC4_seq2_TXT=Not Used  ADC4_seq2_align=Right aligned  ADC4_seq2_overSampling=x1 (12 bits)  ADC5_seq2_TXT=Not Used  ADC5_seq2_align=Right aligned  ADC5_seq2_overSampling=x1 (12 bits)  ADC1_seq2_1_TXT=Not Used  ADC1_seq2_1_align=Right aligned  ADC1_seq2_1_overSampling=x1 (12 bits)  ADC2_seq2_1_TXT=Not Used  ADC2_seq2_1_align=Right aligned  ADC2_seq2_1_overSampling=x1 (12 bits)  ADC3_seq2_1_TXT=Not Used  ADC3_seq2_1_align=Right aligned  ADC3_seq2_1_overSampling=x1 (12 bits)  ADC4_seq2_1_TXT=Not Used  ADC4_seq2_1_align=Right aligned  ADC4_seq2_1_overSampling=x1 (12 bits)  ADC5_seq2_1_TXT=Not Used  ADC5_seq2_1_align=Right aligned  ADC5_seq2_1_overSampling=x1 (12 bits)  ADC1_seq2_2_TXT=Not Used  ADC1_seq2_2_align=Right aligned  ADC1_seq2_2_overSampling=x1 (12 bits)  ADC2_seq2_2_TXT=Not Used  ADC2_seq2_2_align=Right aligned  ADC2_seq2_2_overSampling=x1 (12 bits)  ADC3_seq2_2_TXT=Not Used  ADC3_seq2_2_align=Right aligned  ADC3_seq2_2_overSampling=x1 (12 bits)  ADC4_seq2_2_TXT=Not Used  ADC4_seq2_2_align=Right aligned  ADC4_seq2_2_overSampling=x1 (12 bits)  ADC5_seq2_2_TXT=Not Used  ADC5_seq2_2_align=Right aligned  ADC5_seq2_2_overSampling=x1 (12 bits)  ADC1_seq2_3_TXT=Not Used  ADC1_seq2_3_align=Right aligned  ADC1_seq2_3_overSampling=x1 (12 bits)  ADC2_seq2_3_TXT=Not Used  ADC2_seq2_3_align=Right aligned  ADC2_seq2_3_overSampling=x1 (12 bits)  ADC3_seq2_3_TXT=Not Used  ADC3_seq2_3_align=Right aligned  ADC3_seq2_3_overSampling=x1 (12 bits)  ADC4_seq2_3_TXT=Not Used  ADC4_seq2_3_align=Right aligned  ADC4_seq2_3_overSampling=x1 (12 bits)  ADC5_seq2_3_TXT=Not Used  ADC5_seq2_3_align=Right aligned  ADC5_seq2_3_overSampling=x1 (12 bits)  ADC1_seq2_4_TXT=Not Used  ADC1_seq2_4_align=Right aligned  ADC1_seq2_4_overSampling=x1 (12 bits)  ADC2_seq2_4_TXT=Not Used  ADC2_seq2_4_align=Right aligned  ADC2_seq2_4_overSampling=x1 (12 bits)  ADC3_seq2_4_TXT=Not Used  ADC3_seq2_4_align=Right aligned  ADC3_seq2_4_overSampling=x1 (12 bits)  ADC4_seq2_4_TXT=Not Used  ADC4_seq2_4_align=Right aligned  ADC4_seq2_4_overSampling=x1 (12 bits)  ADC5_seq2_4_TXT=Not Used  ADC5_seq2_4_align=Right aligned  ADC5_seq2_4_overSampling=x1 (12 bits)  ADC1_seq2_5_TXT=Not Used  ADC1_seq2_5_align=Right aligned  ADC1_seq2_5_overSampling=x1 (12 bits)  ADC2_seq2_5_TXT=Not Used  ADC2_seq2_5_align=Right aligned  ADC2_seq2_5_overSampling=x1 (12 bits)  ADC3_seq2_5_TXT=Not Used  ADC3_seq2_5_align=Right aligned  ADC3_seq2_5_overSampling=x1 (12 bits)  ADC4_seq2_5_TXT=Not Used  ADC4_seq2_5_align=Right aligned  ADC4_seq2_5_overSampling=x1 (12 bits)  ADC5_seq2_5_TXT=Not Used  ADC5_seq2_5_align=Right aligned  ADC5_seq2_5_overSampling=x1 (12 bits)  ADC_TRG2_ACCBRST_seq2=Burst - not interruptible  ADC1_NINSEL_seq2_TXT=Vss - single ended (unsigned)  ADC2_NINSEL_seq2_TXT=Vss - single ended (unsigned)  ADC3_NINSEL_seq2_TXT=Vss - single ended (unsigned)  ADC4_NINSEL_seq2_TXT=Vss - single ended (unsigned)  ADC5_NINSEL_seq2_TXT=Vss - single ended (unsigned)  TrigTimeStep_seq2=off  info_seq2=0  TrigSource_seq3_TXT=after previous sequence  SampleTime_seq3_Tad_TXT="0.5 Tad  = 6.25ns  -  Rin < 0 kOhm"  ADC1_seq3_TXT=Not Used  ADC1_seq3_align=Right aligned  ADC1_seq3_overSampling=x1 (12 bits)  ADC2_seq3_TXT=Not Used  ADC2_seq3_align=Right aligned  ADC2_seq3_overSampling=x1 (12 bits)  ADC3_seq3_TXT=Not Used  ADC3_seq3_align=Right aligned  ADC3_seq3_overSampling=x1 (12 bits)  ADC4_seq3_TXT=Not Used  ADC4_seq3_align=Right aligned  ADC4_seq3_overSampling=x1 (12 bits)  ADC5_seq3_TXT=Not Used  ADC5_seq3_align=Right aligned  ADC5_seq3_overSampling=x1 (12 bits)  ADC1_seq3_1_TXT=Not Used  ADC1_seq3_1_align=Right aligned  ADC1_seq3_1_overSampling=x1 (12 bits)  ADC2_seq3_1_TXT=Not Used  ADC2_seq3_1_align=Right aligned  ADC2_seq3_1_overSampling=x1 (12 bits)  ADC3_seq3_1_TXT=Not Used  ADC3_seq3_1_align=Right aligned  ADC3_seq3_1_overSampling=x1 (12 bits)  ADC4_seq3_1_TXT=Not Used  ADC4_seq3_1_align=Right aligned  ADC4_seq3_1_overSampling=x1 (12 bits)  ADC5_seq3_1_TXT=Not Used  ADC5_seq3_1_align=Right aligned  ADC5_seq3_1_overSampling=x1 (12 bits)  ADC1_seq3_2_TXT=Not Used  ADC1_seq3_2_align=Right aligned  ADC1_seq3_2_overSampling=x1 (12 bits)  ADC2_seq3_2_TXT=Not Used  ADC2_seq3_2_align=Right aligned  ADC2_seq3_2_overSampling=x1 (12 bits)  ADC3_seq3_2_TXT=Not Used  ADC3_seq3_2_align=Right aligned  ADC3_seq3_2_overSampling=x1 (12 bits)  ADC4_seq3_2_TXT=Not Used  ADC4_seq3_2_align=Right aligned  ADC4_seq3_2_overSampling=x1 (12 bits)  ADC5_seq3_2_TXT=Not Used  ADC5_seq3_2_align=Right aligned  ADC5_seq3_2_overSampling=x1 (12 bits)  ADC1_seq3_3_TXT=Not Used  ADC1_seq3_3_align=Right aligned  ADC1_seq3_3_overSampling=x1 (12 bits)  ADC2_seq3_3_TXT=Not Used  ADC2_seq3_3_align=Right aligned  ADC2_seq3_3_overSampling=x1 (12 bits)  ADC3_seq3_3_TXT=Not Used  ADC3_seq3_3_align=Right aligned  ADC3_seq3_3_overSampling=x1 (12 bits)  ADC4_seq3_3_TXT=Not Used  ADC4_seq3_3_align=Right aligned  ADC4_seq3_3_overSampling=x1 (12 bits)  ADC5_seq3_3_TXT=Not Used  ADC5_seq3_3_align=Right aligned  ADC5_seq3_3_overSampling=x1 (12 bits)  ADC1_seq3_4_TXT=Not Used  ADC1_seq3_4_align=Right aligned  ADC1_seq3_4_overSampling=x1 (12 bits)  ADC2_seq3_4_TXT=Not Used  ADC2_seq3_4_align=Right aligned  ADC2_seq3_4_overSampling=x1 (12 bits)  ADC3_seq3_4_TXT=Not Used  ADC3_seq3_4_align=Right aligned  ADC3_seq3_4_overSampling=x1 (12 bits)  ADC4_seq3_4_TXT=Not Used  ADC4_seq3_4_align=Right aligned  ADC4_seq3_4_overSampling=x1 (12 bits)  ADC5_seq3_4_TXT=Not Used  ADC5_seq3_4_align=Right aligned  ADC5_seq3_4_overSampling=x1 (12 bits)  ADC1_seq3_5_TXT=Not Used  ADC1_seq3_5_align=Right aligned  ADC1_seq3_5_overSampling=x1 (12 bits)  ADC2_seq3_5_TXT=Not Used  ADC2_seq3_5_align=Right aligned  ADC2_seq3_5_overSampling=x1 (12 bits)  ADC3_seq3_5_TXT=Not Used  ADC3_seq3_5_align=Right aligned  ADC3_seq3_5_overSampling=x1 (12 bits)  ADC4_seq3_5_TXT=Not Used  ADC4_seq3_5_align=Right aligned  ADC4_seq3_5_overSampling=x1 (12 bits)  ADC5_seq3_5_TXT=Not Used  ADC5_seq3_5_align=Right aligned  ADC5_seq3_5_overSampling=x1 (12 bits)  ADC_TRG2_ACCBRST_seq3=Burst - not interruptible  ADC1_NINSEL_seq3_TXT=Vss - single ended (unsigned)  ADC2_NINSEL_seq3_TXT=Vss - single ended (unsigned)  ADC3_NINSEL_seq3_TXT=Vss - single ended (unsigned)  ADC4_NINSEL_seq3_TXT=Vss - single ended (unsigned)  ADC5_NINSEL_seq3_TXT=Vss - single ended (unsigned)  TrigTimeStep_seq3=off  info_seq3=0  TrigSource_seq4_TXT=after previous sequence  SampleTime_seq4_Tad_TXT="0.5 Tad  = 6.25ns  -  Rin < 0 kOhm"  ADC1_seq4_TXT=Not Used  ADC1_seq4_align=Right aligned  ADC1_seq4_overSampling=x1 (12 bits)  ADC2_seq4_TXT=Not Used  ADC2_seq4_align=Right aligned  ADC2_seq4_overSampling=x1 (12 bits)  ADC3_seq4_TXT=Not Used  ADC3_seq4_align=Right aligned  ADC3_seq4_overSampling=x1 (12 bits)  ADC4_seq4_TXT=Not Used  ADC4_seq4_align=Right aligned  ADC4_seq4_overSampling=x1 (12 bits)  ADC5_seq4_TXT=Not Used  ADC5_seq4_align=Right aligned  ADC5_seq4_overSampling=x1 (12 bits)  ADC1_seq4_1_TXT=Not Used  ADC1_seq4_1_align=Right aligned  ADC1_seq4_1_overSampling=x1 (12 bits)  ADC2_seq4_1_TXT=Not Used  ADC2_seq4_1_align=Right aligned  ADC2_seq4_1_overSampling=x1 (12 bits)  ADC3_seq4_1_TXT=Not Used  ADC3_seq4_1_align=Right aligned  ADC3_seq4_1_overSampling=x1 (12 bits)  ADC4_seq4_1_TXT=Not Used  ADC4_seq4_1_align=Right aligned  ADC4_seq4_1_overSampling=x1 (12 bits)  ADC5_seq4_1_TXT=Not Used  ADC5_seq4_1_align=Right aligned  ADC5_seq4_1_overSampling=x1 (12 bits)  ADC1_seq4_2_TXT=Not Used  ADC1_seq4_2_align=Right aligned  ADC1_seq4_2_overSampling=x1 (12 bits)  ADC2_seq4_2_TXT=Not Used  ADC2_seq4_2_align=Right aligned  ADC2_seq4_2_overSampling=x1 (12 bits)  ADC3_seq4_2_TXT=Not Used  ADC3_seq4_2_align=Right aligned  ADC3_seq4_2_overSampling=x1 (12 bits)  ADC4_seq4_2_TXT=Not Used  ADC4_seq4_2_align=Right aligned  ADC4_seq4_2_overSampling=x1 (12 bits)  ADC5_seq4_2_TXT=Not Used  ADC5_seq4_2_align=Right aligned  ADC5_seq4_2_overSampling=x1 (12 bits)  ADC1_seq4_3_TXT=Not Used  ADC1_seq4_3_align=Right aligned  ADC1_seq4_3_overSampling=x1 (12 bits)  ADC2_seq4_3_TXT=Not Used  ADC2_seq4_3_align=Right aligned  ADC2_seq4_3_overSampling=x1 (12 bits)  ADC3_seq4_3_TXT=Not Used  ADC3_seq4_3_align=Right aligned  ADC3_seq4_3_overSampling=x1 (12 bits)  ADC4_seq4_3_TXT=Not Used  ADC4_seq4_3_align=Right aligned  ADC4_seq4_3_overSampling=x1 (12 bits)  ADC5_seq4_3_TXT=Not Used  ADC5_seq4_3_align=Right aligned  ADC5_seq4_3_overSampling=x1 (12 bits)  ADC1_seq4_4_TXT=Not Used  ADC1_seq4_4_align=Right aligned  ADC1_seq4_4_overSampling=x1 (12 bits)  ADC2_seq4_4_TXT=Not Used  ADC2_seq4_4_align=Right aligned  ADC2_seq4_4_overSampling=x1 (12 bits)  ADC3_seq4_4_TXT=Not Used  ADC3_seq4_4_align=Right aligned  ADC3_seq4_4_overSampling=x1 (12 bits)  ADC4_seq4_4_TXT=Not Used  ADC4_seq4_4_align=Right aligned  ADC4_seq4_4_overSampling=x1 (12 bits)  ADC5_seq4_4_TXT=Not Used  ADC5_seq4_4_align=Right aligned  ADC5_seq4_4_overSampling=x1 (12 bits)  ADC1_seq4_5_TXT=Not Used  ADC1_seq4_5_align=Right aligned  ADC1_seq4_5_overSampling=x1 (12 bits)  ADC2_seq4_5_TXT=Not Used  ADC2_seq4_5_align=Right aligned  ADC2_seq4_5_overSampling=x1 (12 bits)  ADC3_seq4_5_TXT=Not Used  ADC3_seq4_5_align=Right aligned  ADC3_seq4_5_overSampling=x1 (12 bits)  ADC4_seq4_5_TXT=Not Used  ADC4_seq4_5_align=Right aligned  ADC4_seq4_5_overSampling=x1 (12 bits)  ADC5_seq4_5_TXT=Not Used  ADC5_seq4_5_align=Right aligned  ADC5_seq4_5_overSampling=x1 (12 bits)  ADC_TRG2_ACCBRST_seq4=Burst - not interruptible  ADC1_NINSEL_seq4_TXT=Vss - single ended (unsigned)  ADC2_NINSEL_seq4_TXT=Vss - single ended (unsigned)  ADC3_NINSEL_seq4_TXT=Vss - single ended (unsigned)  ADC4_NINSEL_seq4_TXT=Vss - single ended (unsigned)  ADC5_NINSEL_seq4_TXT=Vss - single ended (unsigned)  TrigTimeStep_seq4=off  info_seq4=0  TrigSource_seq5_TXT=after previous sequence  SampleTime_seq5_Tad_TXT="0.5 Tad  = 6.25ns  -  Rin < 0 kOhm"  ADC1_seq5_TXT=Not Used  ADC1_seq5_align=Right aligned  ADC1_seq5_overSampling=x1 (12 bits)  ADC2_seq5_TXT=Not Used  ADC2_seq5_align=Right aligned  ADC2_seq5_overSampling=x1 (12 bits)  ADC3_seq5_TXT=Not Used  ADC3_seq5_align=Right aligned  ADC3_seq5_overSampling=x1 (12 bits)  ADC4_seq5_TXT=Not Used  ADC4_seq5_align=Right aligned  ADC4_seq5_overSampling=x1 (12 bits)  ADC5_seq5_TXT=Not Used  ADC5_seq5_align=Right aligned  ADC5_seq5_overSampling=x1 (12 bits)  ADC1_seq5_1_TXT=Not Used  ADC1_seq5_1_align=Right aligned  ADC1_seq5_1_overSampling=x1 (12 bits)  ADC2_seq5_1_TXT=Not Used  ADC2_seq5_1_align=Right aligned  ADC2_seq5_1_overSampling=x1 (12 bits)  ADC3_seq5_1_TXT=Not Used  ADC3_seq5_1_align=Right aligned  ADC3_seq5_1_overSampling=x1 (12 bits)  ADC4_seq5_1_TXT=Not Used  ADC4_seq5_1_align=Right aligned  ADC4_seq5_1_overSampling=x1 (12 bits)  ADC5_seq5_1_TXT=Not Used  ADC5_seq5_1_align=Right aligned  ADC5_seq5_1_overSampling=x1 (12 bits)  ADC1_seq5_2_TXT=Not Used  ADC1_seq5_2_align=Right aligned  ADC1_seq5_2_overSampling=x1 (12 bits)  ADC2_seq5_2_TXT=Not Used  ADC2_seq5_2_align=Right aligned  ADC2_seq5_2_overSampling=x1 (12 bits)  ADC3_seq5_2_TXT=Not Used  ADC3_seq5_2_align=Right aligned  ADC3_seq5_2_overSampling=x1 (12 bits)  ADC4_seq5_2_TXT=Not Used  ADC4_seq5_2_align=Right aligned  ADC4_seq5_2_overSampling=x1 (12 bits)  ADC5_seq5_2_TXT=Not Used  ADC5_seq5_2_align=Right aligned  ADC5_seq5_2_overSampling=x1 (12 bits)  ADC1_seq5_3_TXT=Not Used  ADC1_seq5_3_align=Right aligned  ADC1_seq5_3_overSampling=x1 (12 bits)  ADC2_seq5_3_TXT=Not Used  ADC2_seq5_3_align=Right aligned  ADC2_seq5_3_overSampling=x1 (12 bits)  ADC3_seq5_3_TXT=Not Used  ADC3_seq5_3_align=Right aligned  ADC3_seq5_3_overSampling=x1 (12 bits)  ADC4_seq5_3_TXT=Not Used  ADC4_seq5_3_align=Right aligned  ADC4_seq5_3_overSampling=x1 (12 bits)  ADC5_seq5_3_TXT=Not Used  ADC5_seq5_3_align=Right aligned  ADC5_seq5_3_overSampling=x1 (12 bits)  ADC1_seq5_4_TXT=Not Used  ADC1_seq5_4_align=Right aligned  ADC1_seq5_4_overSampling=x1 (12 bits)  ADC2_seq5_4_TXT=Not Used  ADC2_seq5_4_align=Right aligned  ADC2_seq5_4_overSampling=x1 (12 bits)  ADC3_seq5_4_TXT=Not Used  ADC3_seq5_4_align=Right aligned  ADC3_seq5_4_overSampling=x1 (12 bits)  ADC4_seq5_4_TXT=Not Used  ADC4_seq5_4_align=Right aligned  ADC4_seq5_4_overSampling=x1 (12 bits)  ADC5_seq5_4_TXT=Not Used  ADC5_seq5_4_align=Right aligned  ADC5_seq5_4_overSampling=x1 (12 bits)  ADC1_seq5_5_TXT=Not Used  ADC1_seq5_5_align=Right aligned  ADC1_seq5_5_overSampling=x1 (12 bits)  ADC2_seq5_5_TXT=Not Used  ADC2_seq5_5_align=Right aligned  ADC2_seq5_5_overSampling=x1 (12 bits)  ADC3_seq5_5_TXT=Not Used  ADC3_seq5_5_align=Right aligned  ADC3_seq5_5_overSampling=x1 (12 bits)  ADC4_seq5_5_TXT=Not Used  ADC4_seq5_5_align=Right aligned  ADC4_seq5_5_overSampling=x1 (12 bits)  ADC5_seq5_5_TXT=Not Used  ADC5_seq5_5_align=Right aligned  ADC5_seq5_5_overSampling=x1 (12 bits)  ADC_TRG2_ACCBRST_seq5=Burst - not interruptible  ADC1_NINSEL_seq5_TXT=Vss - single ended (unsigned)  ADC2_NINSEL_seq5_TXT=Vss - single ended (unsigned)  ADC3_NINSEL_seq5_TXT=Vss - single ended (unsigned)  ADC4_NINSEL_seq5_TXT=Vss - single ended (unsigned)  ADC5_NINSEL_seq5_TXT=Vss - single ended (unsigned)  TrigTimeStep_seq5=off  info_seq5=0
      settings: SourceProductName=MPLAB Device Blocks for Simulink
  Ia : Outport  VectorParamsAs1DForOutWhenUnconnected=off
  Ib : Outport  Port=2  VectorParamsAs1DForOutWhenUnconnected=off
  IBus : Outport  Port=3  VectorParamsAs1DForOutWhenUnconnected=off
  Pot : Outport  Port=4  VectorParamsAs1DForOutWhenUnconnected=off
  V_BUS : Outport  Port=5  VectorParamsAs1DForOutWhenUnconnected=off
  iL : Outport  Port=6  VectorParamsAs1DForOutWhenUnconnected=off
  Vac : Outport  Port=7  VectorParamsAs1DForOutWhenUnconnected=off
  wires:
  ADC HS 12b dsPICA/1 -> V_BUS/1
  ADC HS 12b dsPICA/3 -> iL/1
  ADC HS 12b dsPICA/2 -> Vac/1
  ADC HS 12b dsPICA1/3 -> Pot/1
  ADC HS 12b dsPICA1/1 -> Ia/1
  ADC HS 12b dsPICA1/2 -> Ib/1
  ADC HS 12b dsPICA1/4 -> IBus/1

== system mchp_acim_dsPIC33A/MCHV-230VAC-1.5kW Development Board dsPIC33AK128MC106 MC DIM/Center & sign reversal ==
  Bias Update : Inport
  I_ab : Inport  Port=2
  Average and Sign reverse : Sum  Inputs=+-  OutDataTypeStr=int16  AccumDataTypeStr=int32  SaturateOnIntegerOverflow=on
  Downsample Averaged 2000 samples remove bias : Subsystem  mask{DownSample=2000}
      mask prompts: DownSample "DownSample Factor"
  Rate Transition1 : RateTransition  Deterministic=off
  Iab : Outport
  wires:
  I_ab/1 -> Downsample Averaged 2000 samples remove bias/1(In1), Average and Sign reverse/2  "Iab_raw"
  Bias Update/1 -> Downsample Averaged 2000 samples remove bias/Enable  "Enable"
  Downsample Averaged 2000 samples remove bias/1(Out1) -> Rate Transition1/1
  Average and Sign reverse/1 -> Iab/1  "I_ab"
  Rate Transition1/1 -> Average and Sign reverse/1  "Offset_Value"

== system mchp_acim_dsPIC33A/MCHV-230VAC-1.5kW Development Board dsPIC33AK128MC106 MC DIM/Center & sign reversal1 ==
  iL : Inport
  Bias Update : Inport  Port=2
  Data Type Conversion : DataTypeConversion  OutDataTypeStr=int16  SaturateOnIntegerOverflow=off  RndMeth=Floor
  Moving Average : Subsystem  mask{DownSample=2000, InitialValue=32767}
      mask prompts: DownSample "DownSample Factor"; InitialValue "Initial Value"
      settings: AttributesFormatString=|
      | %<DownSample> Samples
      | Init val: %<InitialValue>
      mask DialogControl InitialValue Tooltip: Output value before first execution of bias removal is completed
  remova bias : Sum  Inputs=+-  OutDataTypeStr=int16  AccumDataTypeStr=int32
  IL : Outport
  wires:
  iL/1 -> Moving Average/1(In1), remova bias/1  "Iab_raw"
  Bias Update/1 -> Moving Average/Enable  "Enable"
  Moving Average/1(Out2) -> Data Type Conversion/1
  remova bias/1 -> IL/1  "iL"
  Data Type Conversion/1 -> remova bias/2  "Offset_Value"

== system mchp_acim_dsPIC33A/MCHV-230VAC-1.5kW Development Board dsPIC33AK128MC106 MC DIM/Downsample Averaged x20 ==
  note: DownSample & Average by changing data scaling
  In1 : Inport
  Compare To Constant : simulink/Logic and Bit Operations/Compare To Constant  relop===  const=1  OutDataTypeStr=boolean
  Counter Limited : simulink/Sources/Counter Limited  uplimit=DownSample-1  tsamp=-1
  Data Type Duplicate : DataTypeDuplicate
  Data Type Propagation : simulink/Signal Attributes/Data Type Propagation  PropDataType=fixdt(1, 16)  IfRefDouble=double  IfRefSingle=single  IsSigned=IsSigned1 or IsSigned2  NumBitsBase=NumBits1+NumBits2  NumBitsMult=1  NumBitsAdd=0  NumBitsAllowFinal=-1  PropScaling=2^-10  ValuesUsedBestPrec=[5 -7]  SlopeBase=Slope1  SlopeMult=1  SlopeAdd=0  BiasBase=Bias1  BiasMult=1  BiasAdd=0
  Data Type Propagation1 : simulink/Signal Attributes/Data Type Propagation  PropDataType=fixdt(1, 16)  IfRefDouble=double  IfRefSingle=single  IsSigned=IsSigned1 or IsSigned2  NumBitsBase=NumBits1+NumBits2  NumBitsMult=1  NumBitsAdd=0  NumBitsAllowFinal=-1  PropScaling=2^-10  ValuesUsedBestPrec=[5 -7]  SlopeBase=PosRange1  SlopeMult=1  SlopeAdd=0  BiasBase=Bias1  BiasMult=1  BiasAdd=0
  Discrete-Time Integrator : DiscreteIntegrator  IntegratorMethod=Accumulation: Backward Euler  gainval=1  ExternalReset=sampled level  SampleTime=-1  OutDataTypeStr=Inherit: Inherit via back propagation  ICPrevOutput=DiscIntNeverNeededParam  ICPrevScaledInput=DiscIntNeverNeededParam
  Gain : Gain  Gain=1/DownSample  OutDataTypeStr=Inherit: Inherit via back propagation  RndMeth=Round
  Gain1 : Gain  Gain=1/DownSample  OutDataTypeStr=Inherit: Inherit via back propagation
  Rate Transition1 : RateTransition  OutPortSampleTimeOpt=Multiple of input port sample time  OutPortSampleTimeMultiple=DownSample  OutPortSampleTime=DownSample
  Rate Transition3 : RateTransition  OutPortSampleTimeOpt=Multiple of input port sample time  OutPortSampleTimeMultiple=DownSample  OutPortSampleTime=DownSample
  Terminator : Terminator
  Out1 : Outport  VectorParamsAs1DForOutWhenUnconnected=off
  wires:
  Gain1/1 -> Data Type Propagation1/3, Terminator/1
  Rate Transition1/1 -> Data Type Duplicate/1, Data Type Propagation1/1, Data Type Propagation1/2
  Gain/1 -> Out1/1, Data Type Duplicate/2
  Counter Limited/1 -> Compare To Constant/1
  Discrete-Time Integrator/1 -> Rate Transition3/1, Data Type Propagation/3
  Compare To Constant/1 -> Discrete-Time Integrator/2
  In1/1 -> Data Type Propagation/1, Data Type Propagation/2, Discrete-Time Integrator/1, Rate Transition1/1
  Rate Transition3/1 -> Gain/1, Gain1/1
